simulink model "Wiper_system"  (R2017b)
settings: Solver=VariableStepAuto  StartTime=0.0  StopTime=7  RelTol=1e-3
undefined symbols (not defined in the file): sigbuilder_block
settings Model: SnapshotBufferSize=1  SnapshotInterval=1  Creator=ECoDe_user19  LastModifiedBy=ECoDe_user11
settings DebuggingCC: SignalInfNanChecking=warning  UniqueDataStoreMsg=warning  StrictBusMsg=ErrorOnBusTreatedAsVector
settings ConfigComp: CovEnable=on  RecordCoverage=on  CovMetricSettings=dcmwe  CovModelRefEnable=on  CovExternalEMLEnable=off  CovSFcnEnable=off

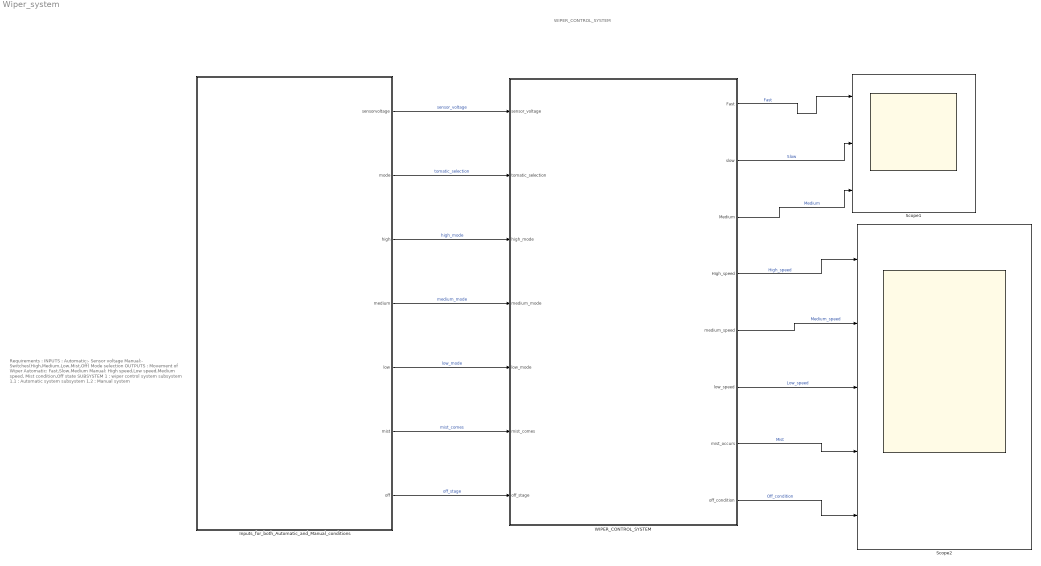
== system Wiper_system ==
  note: WIPER_CONTROL_SYSTEM
  note: Requirements :
      |
      | INPUTS :
      | Automatic:-
      | Sensor voltage
      | Manual:-
      | Switches(High,Medium,Low,Mist,Off)
      |
      | Mode selection
      |
      | OUTPUTS :
      | Movement of Wiper
      | Automatic:
      | Fast,Slow,Medium
      | Manual:
      | High speed,Low speed,Medium speed,
      | Mist condition,Off state
      |
      | SUBSYSTEM 1 :
      | wiper control system
      | subsystem 1.1 :
      | Automatic system
      | subsystem 1.2 :
      | Manual system
  Inputs_for_both_Automatic_and_Manual_conditions : Subsystem  Tag=STV Subsys  LoadFcn=sigbuilder_block('load');  StartFcn=sigbuilder_block('start');  StopFcn=sigbuilder_block('stop');  ClipboardFcn=sigbuilder_block('clipboard');  mask(Sigbuilder block){tuvar=[0:10]}
      mask help: Simulink:masks:SigbuilderBlock_MD
      mask init:
      | if ~strcmp(get_param(bdroot(gcbh),'SimulationStatus'),'stopped') tuvar = sigbuilder_block('maskInit'); end
      settings: CopyFcn=sigbuilder_block('copy');  DeleteFcn=sigbuilder_block('delete');  ModelCloseFcn=sigbuilder_block('modelClose');  PreSaveFcn=sigbuilder_block('preSave');  PauseFcn=sigbuilder_block('pause');  ContinueFcn=sigbuilder_block('continue');  NameChangeFcn=sigbuilder_block('namechange');  OpenFcn=sigbuilder_block('open',[433.5 159 550.5 363.75 ]);  CloseFcn=sigbuilder_block('close');
      mask Display: plot(0, 0, 100, 100,[2, 2, 32, 32, 2], [68, 8, 8, 68, 68],[32, 2], [38, 38], [32, 19, 2],[53, 60, 44], [32, 17, 17, 2],[16, 16, 31, 31]);txt = getActiveGroup(gcbh);text(2, 100, txt,'verticalAlignment', 'top');
  Scope1 : Scope  NumInputPorts=3
  Scope2 : Scope  NumInputPorts=5
  WIPER_CONTROL_SYSTEM : Subsystem
  wires:
  WIPER_CONTROL_SYSTEM/4(High_speed) -> Scope2/1  "High_speed"
  WIPER_CONTROL_SYSTEM/7(mist_occurs) -> Scope2/4  "Mist"
  WIPER_CONTROL_SYSTEM/6(low_speed) -> Scope2/3  "Low_speed"
  WIPER_CONTROL_SYSTEM/5(medium_speed) -> Scope2/2  "Medium_speed"
  WIPER_CONTROL_SYSTEM/8(off_condition) -> Scope2/5  "Off_condition"
  Inputs_for_both_Automatic_and_Manual_conditions/1(sensorvoltage) -> WIPER_CONTROL_SYSTEM/1(sensor_voltage)  "sensor_voltage"
  Inputs_for_both_Automatic_and_Manual_conditions/2(mode) -> WIPER_CONTROL_SYSTEM/2(tomatic_selection)  "tomatic_selection"
  Inputs_for_both_Automatic_and_Manual_conditions/3(high) -> WIPER_CONTROL_SYSTEM/3(high_mode)  "high_mode"
  Inputs_for_both_Automatic_and_Manual_conditions/4(medium) -> WIPER_CONTROL_SYSTEM/4(medium_mode)  "medium_mode"
  Inputs_for_both_Automatic_and_Manual_conditions/5(low) -> WIPER_CONTROL_SYSTEM/5(low_mode)  "low_mode"
  Inputs_for_both_Automatic_and_Manual_conditions/6(mist) -> WIPER_CONTROL_SYSTEM/6(mist_comes)  "mist_comes"
  Inputs_for_both_Automatic_and_Manual_conditions/7(off) -> WIPER_CONTROL_SYSTEM/7(off_stage)  "off_stage"
  WIPER_CONTROL_SYSTEM/1(Fast) -> Scope1/1  "Fast"
  WIPER_CONTROL_SYSTEM/2(slow) -> Scope1/2  "Slow"
  WIPER_CONTROL_SYSTEM/3(Medium) -> Scope1/3  "Medium"

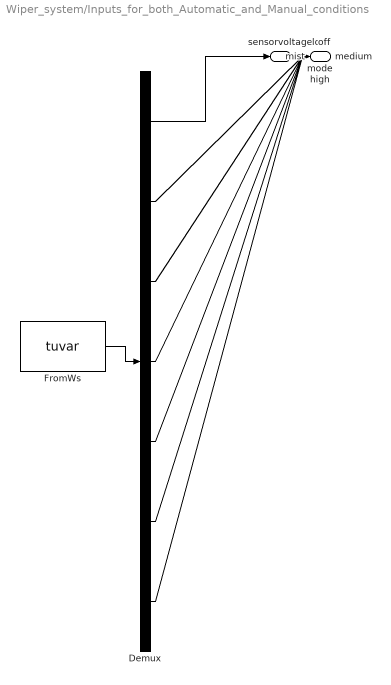
== system Wiper_system/Inputs_for_both_Automatic_and_Manual_conditions ==
  Demux : Demux  Tag=STV Demux  Outputs=7
  FromWs : FromWorkspace  Tag=STV FromWs  VariableName=tuvar  SampleTime=0
      SigBuilderData=|
      | common.afterFinalStr = 'Extrapolate'
      | common.sampleTime = 0
      | dataSet.timeRange = [0 7]
      | dataSet.name = 'Sheet1'
      | sbobj.Name = 'Signal Builder'
      | sbobj.Groups.Name = 'Sheet1'
      | sbobj.Groups.Signals(1).Name = 'sensorvoltage'
      | sbobj.Groups.Signals(1).XData = [0 0.2 0.4 0.6 0.8 1 1.2 1.4 1.6 1.8 2 2.2 2.4 2.6 2.8 3 3.2 3.4 3.6 3.8 4 4.2 4.4 4.6 4.8 5 5.2 5.4 5.6 5.8 6 6.2 6.4 6.6 6.8 7]
      | sbobj.Groups.Signals(1).YData = [0 0.5 1 1.5 2 2.5 3 3.5 4 4.5 5 5.5 6 6.5 7 7.5 8 8.5 9 9.5 10 9 6.3 8 0.4 9.2 3.4 0.8 4 1.2 7 3.4 0.1 9.2 6.4 1.6]
      | sbobj.Groups.Signals(2).Name = 'mode'
      | sbobj.Groups.Signals(2).XData = [0 0.2 0.4 0.6 0.8 1 1.2 1.4 1.6 1.8 2 2.2 2.4 2.6 2.8 3 3.2 3.4 3.6 3.8 4 4.2 4.4 4.6 4.8 5 5.2 5.4 5.6 5.8 6 6.2 6.4 6.6 6.8 7]
      | sbobj.Groups.Signals(2).YData = [0 1 0 1 0 1 1 1 1 1.1 0 1 0 1 0 1 0 1 0 1 0 1 1 0 1 1 0 1 1 0 1 0 1 1 1 1]
      | sbobj.Groups.Signals(3).Name = 'high'
      | sbobj.Groups.Signals(3).XData = [0 0.2 0.4 0.6 0.8 1 1.2 1.4 1.6 1.8 2 2.2 2.4 2.6 2.8 3 3.2 3.4 3.6 3.8 4 4.2 4.4 4.6 4.8 5 5.2 5.4 5.6 5.8 6 6.2 6.4 6.6 6.8 7]
      | sbobj.Groups.Signals(3).YData = [0 0 0 0 1 0 0 0 0 1 0 0 0 0 1 0 0 0 0 1 0 0 0 0 1 0 0 0 0 1 0 0 0 0 1 1]
      | sbobj.Groups.Signals(4).Name = 'medium'
      | sbobj.Groups.Signals(4).XData = [0 0.2 0.4 0.6 0.8 1 1.2 1.4 1.6 1.8 2 2.2 2.4 2.6 2.8 3 3.2 3.4 3.6 3.8 4 4.2 4.4 4.6 4.8 5 5.2 5.4 5.6 5.8 6 6.2 6.4 6.6 6.8 7]
      | sbobj.Groups.Signals(4).YData = [0 0 0 1 0 0 0 0 1 0 0 0 0 1 0 0 0 0 1 0 0 0 0 1 0 0 0 0 1 0 0 0 0 1 0 0]
      | sbobj.Groups.Signals(5).Name = 'low'
      | sbobj.Groups.Signals(5).XData = [0 0.2 0.4 0.6 0.8 1 1.2 1.4 1.6 1.8 2 2.2 2.4 2.6 2.8 3 3.2 3.4 3.6 3.8 4 4.2 4.4 4.6 4.8 5 5.2 5.4 5.6 5.8 6 6.2 6.4 6.6 6.8 7]
      | sbobj.Groups.Signals(5).YData = [0 0 1 0 0 0 0 1 0 0 0 0 1 0 0 0 0 1 0 0 0 0 1 0 0 0 0 1 0 0 0 0 1 0 0 0]
      | sbobj.Groups.Signals(6).Name = 'mist'
      | sbobj.Groups.Signals(6).XData = [0 0.2 0.4 0.6 0.8 1 1.2 1.4 1.6 1.8 2 2.2 2.4 2.6 2.8 3 3.2 3.4 3.6 3.8 4 4.2 4.4 4.6 4.8 5 5.2 5.4 5.6 5.8 6 6.2 6.4 6.6 6.8 7]
      | sbobj.Groups.Signals(6).YData = [0 1 0 0 0 0 1 0 0 0 0 1 0 0 0 0 1 0 0 0 0 1 0 0 0 0 1 0 0 0 0 1 0 0 0 0]
      | sbobj.Groups.Signals(7).Name = 'off'
      | sbobj.Groups.Signals(7).XData = [0 0.2 0.4 0.6 0.8 1 1.2 1.4 1.6 1.8 2 2.2 2.4 2.6 2.8 3 3.2 3.4 3.6 3.8 4 4.2 4.4 4.6 4.8 5 5.2 5.4 5.6 5.8 6 6.2 6.4 6.6 6.8 7]
      | sbobj.Groups.Signals(7).YData = [1 0 0 0 0 1 0 0 0 0 1 0 0 0 0 1 0 0 0 0 1 0 0 0 0 1 0 0 0 0 1 0 0 0 0 0]
      | sbobj.Groups.TimeRange = [0 9.8]
  sensorvoltage : Outport  Tag=STV Outport
  mode : Outport  Tag=STV Outport  Port=2
  high : Outport  Tag=STV Outport  Port=3
  medium : Outport  Tag=STV Outport  Port=4
  low : Outport  Tag=STV Outport  Port=5
  mist : Outport  Tag=STV Outport  Port=6
  off : Outport  Tag=STV Outport  Port=7
  wires:
  Demux/1 -> sensorvoltage/1
  FromWs/1 -> Demux/1
  Demux/2 -> mode/1
  Demux/3 -> high/1
  Demux/4 -> medium/1
  Demux/5 -> low/1
  Demux/6 -> mist/1
  Demux/7 -> off/1

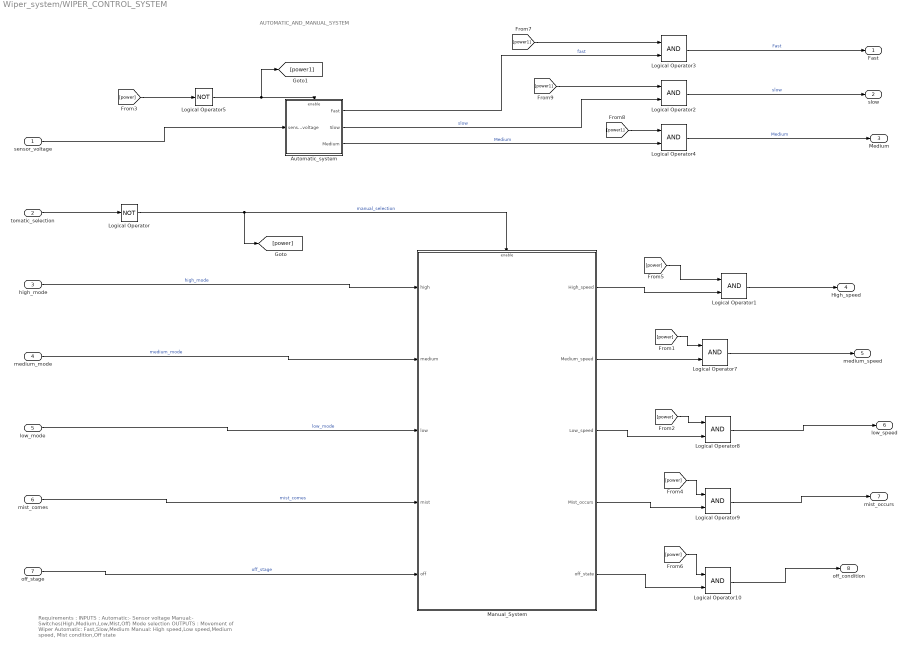
== system Wiper_system/WIPER_CONTROL_SYSTEM ==
  note: AUTOMATIC_AND_MANUAL_SYSTEM
  note: Requirements :
      |
      | INPUTS :
      | Automatic:-
      | Sensor voltage
      | Manual:-
      | Switches(High,Medium,Low,Mist,Off)
      |
      | Mode selection
      |
      | OUTPUTS :
      | Movement of Wiper
      | Automatic:
      | Fast,Slow,Medium
      | Manual:
      | High speed,Low speed,Medium speed,
      | Mist condition,Off state
  sensor_voltage : Inport
  tomatic_selection : Inport  Port=2
  high_mode : Inport  Port=3
  medium_mode : Inport  Port=4
  low_mode : Inport  Port=5
  mist_comes : Inport  Port=6
  off_stage : Inport  Port=7
  Automatic_system : Subsystem
  Logical Operator : Logic  Operator=NOT  AllPortsSameDT=off  OutDataTypeStr=boolean
  Logical Operator{1..4,7..10} (8 alike) : Logic  AllPortsSameDT=off  OutDataTypeStr=boolean
  Logical Operator5 : Logic  Operator=NOT  AllPortsSameDT=off  OutDataTypeStr=boolean
  Manual_System : Subsystem
  Fast : Outport
  slow : Outport  Port=2
  Medium : Outport  Port=3
  High_speed : Outport  Port=4
  medium_speed : Outport  Port=5
  low_speed : Outport  Port=6
  mist_occurs : Outport  Port=7
  off_condition : Outport  Port=8
  wires:
  tomatic_selection/1 -> Logical Operator/1
  Manual_System/5(off_state) -> Logical Operator10/2
  [power] -> Logical Operator7/1
  medium_mode/1 -> Manual_System/2(medium)  "medium_mode"
  Logical Operator1/1 -> High_speed/1
  Logical Operator10/1 -> off_condition/1
  Logical Operator9/1 -> mist_occurs/1
  Logical Operator7/1 -> medium_speed/1
  [power] -> Logical Operator8/1
  low_mode/1 -> Manual_System/3(low)  "low_mode"
  mist_comes/1 -> Manual_System/4(mist)  "mist_comes"
  Logical Operator8/1 -> low_speed/1
  Manual_System/3(Low_speed) -> Logical Operator8/2
  Manual_System/1(High_speed) -> Logical Operator1/2
  off_stage/1 -> Manual_System/5(off)  "off_stage"
  [power] -> Logical Operator10/1
  [power] -> Logical Operator1/1
  [power] -> Logical Operator5/1
  Logical Operator/1 -> [power], Manual_System/Enable  "manual_selection"
  Manual_System/4(Mist_occurs) -> Logical Operator9/2
  Manual_System/2(Medium_speed) -> Logical Operator7/2
  [power] -> Logical Operator9/1
  Logical Operator5/1 -> [power1], Automatic_system/Enable
  high_mode/1 -> Manual_System/1(high)  "high_mode"
  sensor_voltage/1 -> Automatic_system/1(sensorvoltage)
  Automatic_system/1(Fast) -> Logical Operator3/2  "fast"
  Automatic_system/2(Slow) -> Logical Operator2/2  "slow"
  Automatic_system/3(Medium) -> Logical Operator4/2  "Medium"
  [power1] -> Logical Operator3/1
  [power1] -> Logical Operator2/1
  [power1] -> Logical Operator4/1
  Logical Operator3/1 -> Fast/1  "Fast"
  Logical Operator2/1 -> slow/1  "slow"
  Logical Operator4/1 -> Medium/1  "Medium"

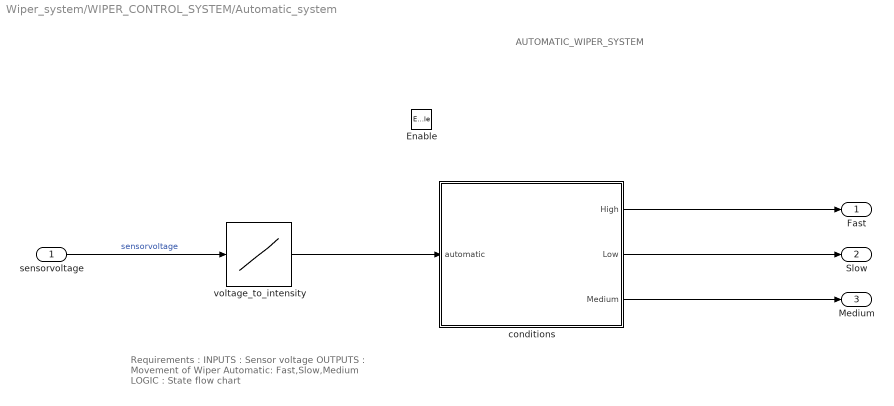
== system Wiper_system/WIPER_CONTROL_SYSTEM/Automatic_system ==
  note: AUTOMATIC_WIPER_SYSTEM
  note: Requirements :
      |
      | INPUTS :
      | Sensor voltage
      |
      | OUTPUTS :
      | Movement of Wiper
      | Automatic:
      | Fast,Slow,Medium
      |
      | LOGIC :
      | State flow chart
  sensorvoltage : Inport
  Enable : EnablePort
  conditions : Stateflow chart  TreatAsAtomicUnit=on
  voltage_to_intensity : Lookup_n-D  NumberOfTableDimensions=1  BreakpointsForDimension1=[0 10]  Table=[40 130]  InternalRulePriority=Speed  RndMeth=Simplest  InputSameDT=on
      settings: AttributesFormatString=%<RndMeth>
  Fast : Outport
  Slow : Outport  Port=2
  Medium : Outport  Port=3
  wires:
  voltage_to_intensity/1 -> conditions/1(automatic)
  conditions/1(High) -> Fast/1
  conditions/2(Low) -> Slow/1
  conditions/3(Medium) -> Medium/1
  sensorvoltage/1 -> voltage_to_intensity/1  "sensorvoltage"

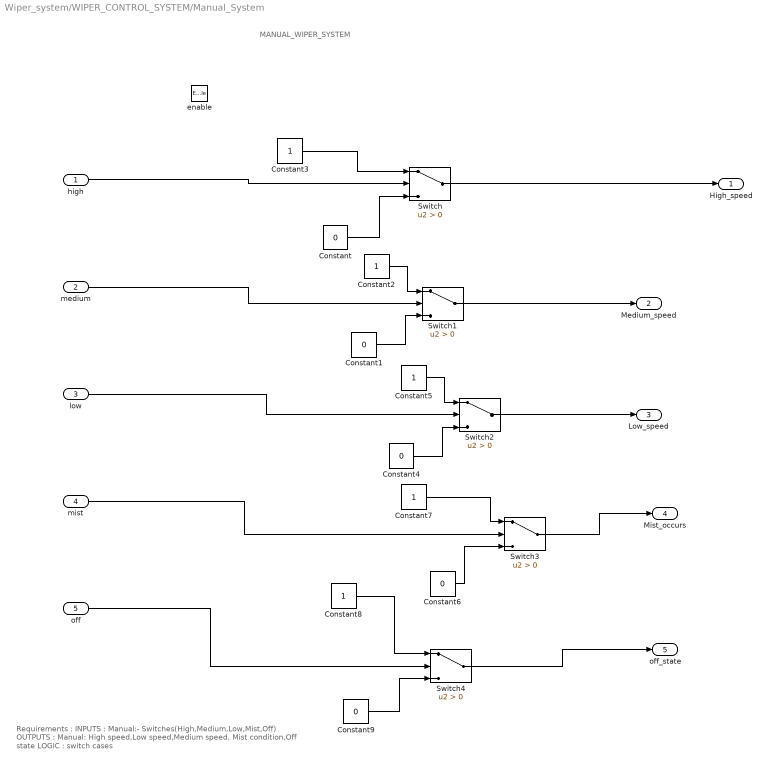
== system Wiper_system/WIPER_CONTROL_SYSTEM/Manual_System ==
  note: MANUAL_WIPER_SYSTEM
  note: Requirements :
      |
      | INPUTS :
      | Manual:-
      | Switches(High,Medium,Low,Mist,Off)
      |
      | OUTPUTS :
      | Manual:
      | High speed,Low speed,Medium speed,
      | Mist condition,Off state
      |
      | LOGIC :
      | switch cases
  high : Inport
  medium : Inport  Port=2
  low : Inport  Port=3
  mist : Inport  Port=4
  off : Inport  Port=5
  enable : EnablePort
  Constant{,1,4,6,9} (5 alike) : Constant  Value=0
  Constant{2..3,5,7..8} (5 alike) : Constant
  Switch{,1..4} (5 alike) : Switch  Criteria=u2 > Threshold
  High_speed : Outport
  Medium_speed : Outport  Port=2
  Low_speed : Outport  Port=3
  Mist_occurs : Outport  Port=4
  off_state : Outport  Port=5
  wires:
  mist/1 -> Switch3/2
  Switch1/1 -> Medium_speed/1
  Constant7/1 -> Switch3/1
  Constant6/1 -> Switch3/3
  Constant/1 -> Switch/3
  Constant8/1 -> Switch4/1
  Constant3/1 -> Switch/1
  Constant5/1 -> Switch2/1
  Constant2/1 -> Switch1/1
  medium/1 -> Switch1/2
  Constant4/1 -> Switch2/3
  Constant9/1 -> Switch4/3
  Constant1/1 -> Switch1/3
  Switch/1 -> High_speed/1
  Switch2/1 -> Low_speed/1
  low/1 -> Switch2/2
  off/1 -> Switch4/2
  Switch4/1 -> off_state/1
  Switch3/1 -> Mist_occurs/1
  high/1 -> Switch/2

== stateflow chart Wiper_system/WIPER_CONTROL_SYSTEM/Automatic_system/conditions ==
  (default) -> (junction 1) : {initial=0}
  (junction 1) -> (junction 5) [order 2] : [automatic>=40 & automatic<70]{Low=1,High=0,Medium=0}
  (junction 1) -> (junction 6) [order 3] : [automatic>=100 & automatic<=130]{High=1,Low=0,Medium=0}
  (junction 1) -> (junction 3) [order 1] : [automatic>=70 & automatic<100]{Medium=1,Low=0,High=0}
  (junction 5) -> (junction 22)
  (junction 6) -> (junction 22)
  (junction 3) -> (junction 22)
  data: automatic input; High output; Low output; Medium output; initial local
